simulink model "observer_sim"  (R2020a)
settings: Solver=VariableStepAuto  StartTime=0.0  StopTime=simulation.stopTime  RelTol=1e-3
values from neighbouring files (symbols this model uses):
  L1 = 1    [Main.m]
  L2 = -0.5    [Main.m]
  MaxCrossings = 3    [Main.m]
  TE = 50    [Main.m]
  Threshold = 0.1    [Main.m]
  tp = 1/(2*pi)    (= 0.159154943092)    [Main.m]
undefined symbols (not defined in the file or in its folder): DiscIntNeverNeededParam, servoModel, simulation
libraries: dspsigops x2, mcbcontrolslib x1, simulink x1
settings Model: Creator=FawadFarooq  LastModifiedBy=FawaD KhaN
settings DebuggingCC: SFMachineParentedDataDiag=error

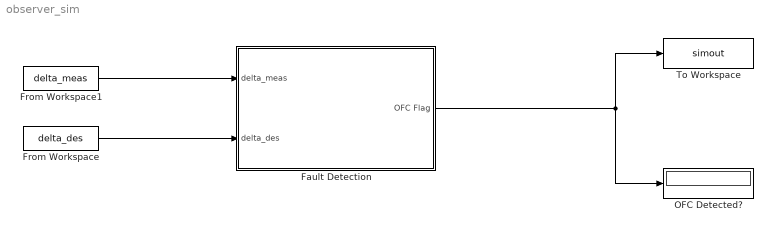
== system observer_sim ==
  Fault Detection : Subsystem
  From Workspace : FromWorkspace  VariableName=delta_des  SampleTime=1/simulation.Fs
  From Workspace1 : FromWorkspace  VariableName=delta_meas  SampleTime=1/simulation.Fs
  OFC Detected? : Display
  To Workspace : ToWorkspace  VariableName=simout  SaveFormat=Timeseries  SampleTime=1/simulation.Fs
  wires:
  Fault Detection/1(OFC Flag) -> OFC Detected?/1, To Workspace/1
  From Workspace1/1 -> Fault Detection/1(delta_meas)
  From Workspace/1 -> Fault Detection/2(delta_des)

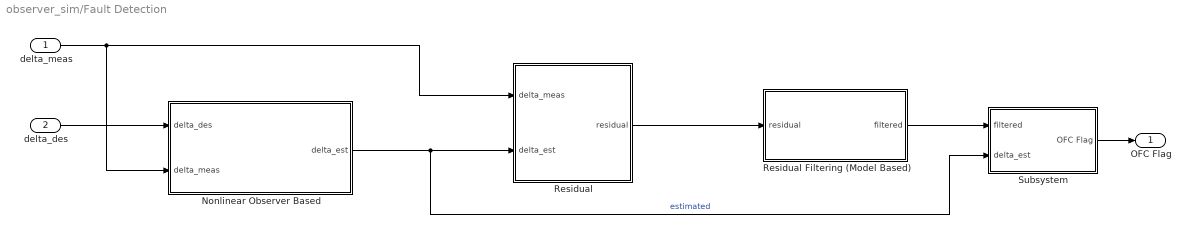
== system observer_sim/Fault Detection ==
  delta_meas : Inport
  delta_des : Inport  Port=2
  Nonlinear Observer Based : Subsystem
  Residual : Subsystem
  Residual Filtering (Model Based) : Subsystem
  Subsystem : Subsystem
  OFC Flag : Outport
  wires:
  Residual/1(residual) -> Residual Filtering (Model Based)/1(residual)
  Nonlinear Observer Based/1(delta_est) -> Subsystem/2(delta_est), Residual/2(delta_est)  "estimated"
  delta_meas/1 -> Nonlinear Observer Based/2(delta_meas), Residual/1(delta_meas)
  Residual Filtering (Model Based)/1(filtered) -> Subsystem/1(filtered)
  delta_des/1 -> Nonlinear Observer Based/1(delta_des)
  Subsystem/1(OFC Flag) -> OFC Flag/1

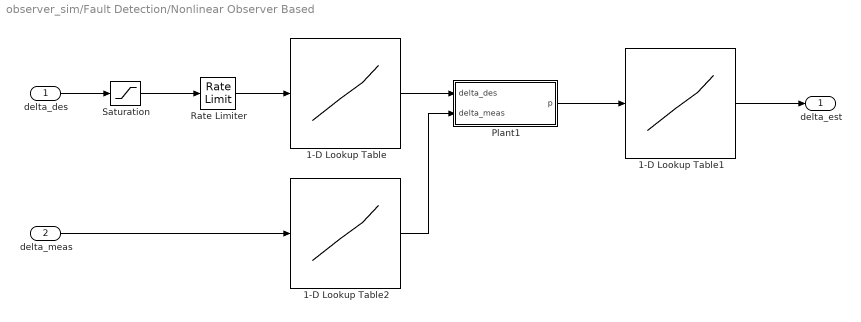
== system observer_sim/Fault Detection/Nonlinear Observer Based ==
  delta_des : Inport
  delta_meas : Inport  Port=2
  1-D Lookup Table : Lookup_n-D  NumberOfTableDimensions=1  BreakpointsForDimension1=[-30,-21,-11,0,14,20]  Table=[77.78,58.55,29.58,0,-37.48,-52.95]  InternalRulePriority=Speed  RndMeth=Simplest  InputSameDT=on
  1-D Lookup Table1 : Lookup_n-D  NumberOfTableDimensions=1  BreakpointsForDimension1=[-52.95, -37.48, 0.0, 29.58, 55.62, 77.78]  Table=[20.0, 14.0, 0.0, -11.0, -21.0, -30.0]  InternalRulePriority=Speed  RndMeth=Simplest  InputSameDT=on
  1-D Lookup Table2 : Lookup_n-D  NumberOfTableDimensions=1  BreakpointsForDimension1=[-30,-21,-11,0,14,20]  Table=[77.78,58.55,29.58,0,-37.48,-52.95]  InternalRulePriority=Speed  RndMeth=Simplest  InputSameDT=on
  Plant1 : Subsystem
  Rate Limiter : RateLimiter  RisingSlewLimit=30  FallingSlewLimit=-30
  Saturation : Saturate  UpperLimit=15  LowerLimit=-30
  delta_est : Outport
  wires:
  Rate Limiter/1 -> 1-D Lookup Table/1
  Saturation/1 -> Rate Limiter/1
  1-D Lookup Table1/1 -> delta_est/1
  delta_des/1 -> Saturation/1
  Plant1/1(p) -> 1-D Lookup Table1/1
  1-D Lookup Table/1 -> Plant1/1(delta_des)
  delta_meas/1 -> 1-D Lookup Table2/1
  1-D Lookup Table2/1 -> Plant1/2(delta_meas)

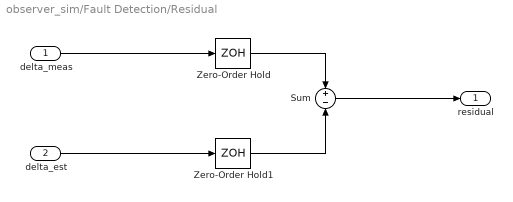
== system observer_sim/Fault Detection/Residual ==
  delta_meas : Inport
  delta_est : Inport  Port=2
  Sum : Sum  Inputs=+|-
  Zero-Order Hold : ZeroOrderHold  SampleTime=1/simulation.Fs
  Zero-Order Hold1 : ZeroOrderHold  SampleTime=1/simulation.Fs
  residual : Outport
  wires:
  Zero-Order Hold/1 -> Sum/1
  delta_meas/1 -> Zero-Order Hold/1
  delta_est/1 -> Zero-Order Hold1/1
  Zero-Order Hold1/1 -> Sum/2
  Sum/1 -> residual/1

== system observer_sim/Fault Detection/Residual Filtering (Model Based) ==
  residual : Inport
  IIR Filter : mcbcontrolslib/IIR Filter  VariantControl=Low Pass Filter  VariantSelect=Low-pass  Filter_constant=0.5  advancedSettings=off  Ts=50e-6  cutOff_freq=3183.0989
      settings: SourceProductBaseCode=MT
  filtered : Outport
  wires:
  IIR Filter/1 -> filtered/1
  residual/1 -> IIR Filter/1

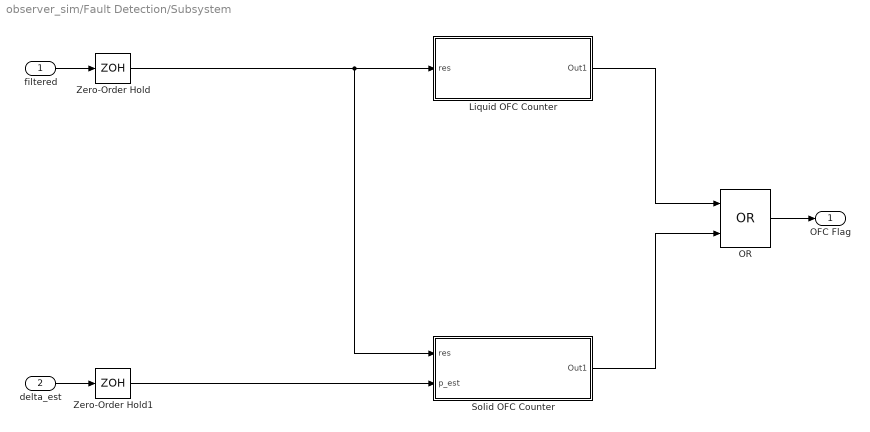
== system observer_sim/Fault Detection/Subsystem ==
  filtered : Inport
  delta_est : Inport  Port=2
  Liquid OFC Counter : Subsystem
  OR : Logic  Operator=OR  IconShape=distinctive  AllPortsSameDT=off  OutDataTypeStr=boolean
  "Solid OFC Counter " : Subsystem
  Zero-Order Hold : ZeroOrderHold  SampleTime=1/simulation.Fs
  Zero-Order Hold1 : ZeroOrderHold  SampleTime=1/simulation.Fs
  OFC Flag : Outport
  wires:
  filtered/1 -> Zero-Order Hold/1
  delta_est/1 -> Zero-Order Hold1/1
  Zero-Order Hold1/1 -> "Solid OFC Counter "/2(p_est)
  Zero-Order Hold/1 -> "Solid OFC Counter "/1(res), Liquid OFC Counter/1(res)
  OR/1 -> OFC Flag/1
  "Solid OFC Counter "/1(Out1) -> OR/2
  Liquid OFC Counter/1(Out1) -> OR/1

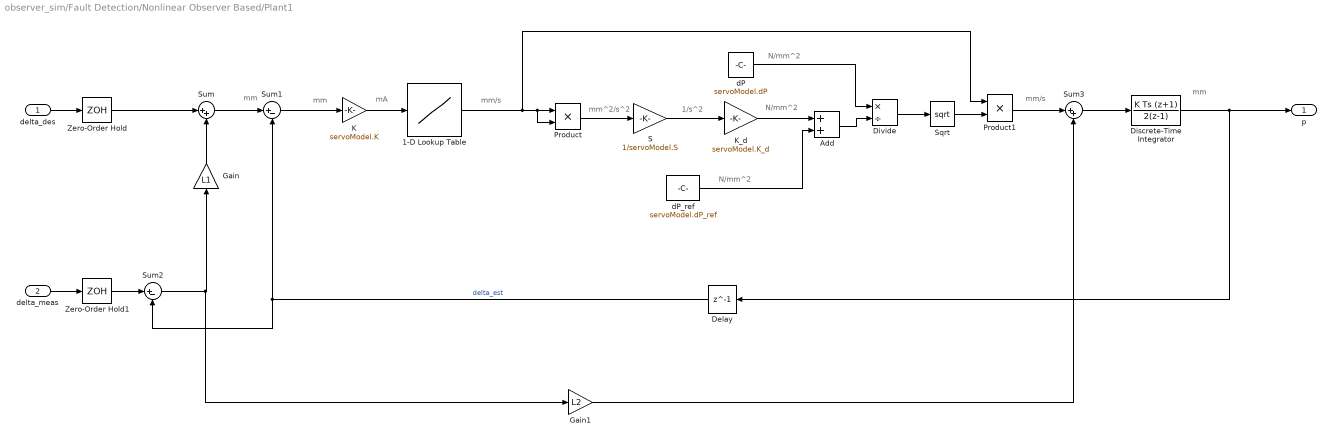
== system observer_sim/Fault Detection/Nonlinear Observer Based/Plant1 ==
  note: N/mm^2
  note: N/mm^2
  note: mm
  note: mA
  note: mm/s
  note: mm^2/s^2
  note: 1/s^2
  note: N/mm^2
  note: mm/s
  note: mm
  note: mm
  delta_des : Inport
  delta_meas : Inport  Port=2
  1-D Lookup Table : Lookup_n-D  NumberOfTableDimensions=1  BreakpointsForDimension1=[-11,-8.45,-2.3,0,2.3,8.45,11]  Table=[-250,-250,-32,0,32,250,250]  InternalRulePriority=Speed  RndMeth=Simplest  InputSameDT=on
  Add : Sum
  Delay : Delay  DelayLength=1  SampleTime=1/simulation.Fs
  Discrete-Time Integrator : DiscreteIntegrator  IntegratorMethod=Integration: Trapezoidal  SampleTime=1/simulation.Fs  ICPrevOutput=DiscIntNeverNeededParam  ICPrevScaledInput=DiscIntNeverNeededParam
  Divide : Product  Inputs=*/
  Gain : Gain  Gain=L1
  Gain1 : Gain  Gain=L2
  K : Gain  Gain=servoModel.K
  K_d : Gain  Gain=servoModel.K_d
  Product : Product
  Product1 : Product
  S : Gain  Gain=1/servoModel.S
  Sqrt : Sqrt  SaturateOnIntegerOverflow=on
  Sum : Sum  Inputs=|++
  Sum1 : Sum  Inputs=|+-
  Sum2 : Sum  Inputs=|+-
  Sum3 : Sum  Inputs=|++
  Zero-Order Hold : ZeroOrderHold  SampleTime=1/simulation.Fs
  Zero-Order Hold1 : ZeroOrderHold  SampleTime=1/simulation.Fs
  dP : Constant  Value=servoModel.dP
  dP_ref : Constant  Value=servoModel.dP_ref
  p : Outport
  wires:
  Delay/1 -> Sum2/2, Sum1/2  "delta_est"
  Discrete-Time Integrator/1 -> p/1, Delay/1
  1-D Lookup Table/1 -> Product1/1, Product/2, Product/1
  dP/1 -> Divide/1
  Sqrt/1 -> Product1/2
  Divide/1 -> Sqrt/1
  S/1 -> K_d/1
  Add/1 -> Divide/2
  K_d/1 -> Add/1
  dP_ref/1 -> Add/2
  Product/1 -> S/1
  K/1 -> 1-D Lookup Table/1
  Sum1/1 -> K/1
  delta_des/1 -> Zero-Order Hold/1
  delta_meas/1 -> Zero-Order Hold1/1
  Zero-Order Hold1/1 -> Sum2/1
  Zero-Order Hold/1 -> Sum/1
  Sum/1 -> Sum1/1
  Gain/1 -> Sum/2
  Product1/1 -> Sum3/1
  Sum3/1 -> Discrete-Time Integrator/1
  Sum2/1 -> Gain1/1, Gain/1
  Gain1/1 -> Sum3/2

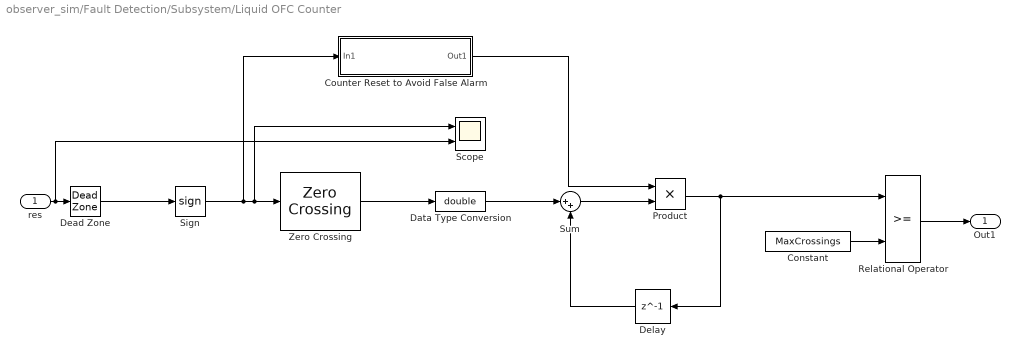
== system observer_sim/Fault Detection/Subsystem/Liquid OFC Counter ==
  res : Inport
  Constant : Constant  Value=MaxCrossings
  Counter Reset to Avoid False Alarm : Subsystem
  Data Type Conversion : DataTypeConversion  OutDataTypeStr=double
  Dead Zone : DeadZone  LowerValue=-Threshold  UpperValue=Threshold  SaturateOnIntegerOverflow=on
  Delay : Delay  DelayLength=1  SampleTime=1/simulation.Fs
  Product : Product
  Relational Operator : RelationalOperator  OutDataTypeStr=boolean  RndMeth=Simplest
  Scope : Scope  NumInputPorts=2
  Sign : Signum
  Sum : Sum  Inputs=|++
  Zero Crossing : dspsigops/Zero Crossing  InputProcessing=Columns as channels (frame based)
      settings: SourceProductBaseCode=DS
  Out1 : Outport
  wires:
  Sum/1 -> Product/2
  Delay/1 -> Sum/2
  Zero Crossing/1 -> Data Type Conversion/1
  Product/1 -> Delay/1, Relational Operator/1
  Relational Operator/1 -> Out1/1
  Sign/1 -> Counter Reset to Avoid False Alarm/1(In1), Scope/1, Zero Crossing/1
  Counter Reset to Avoid False Alarm/1(Out1) -> Product/1
  Dead Zone/1 -> Sign/1
  Data Type Conversion/1 -> Sum/1
  Constant/1 -> Relational Operator/2
  res/1 -> Scope/2, Dead Zone/1

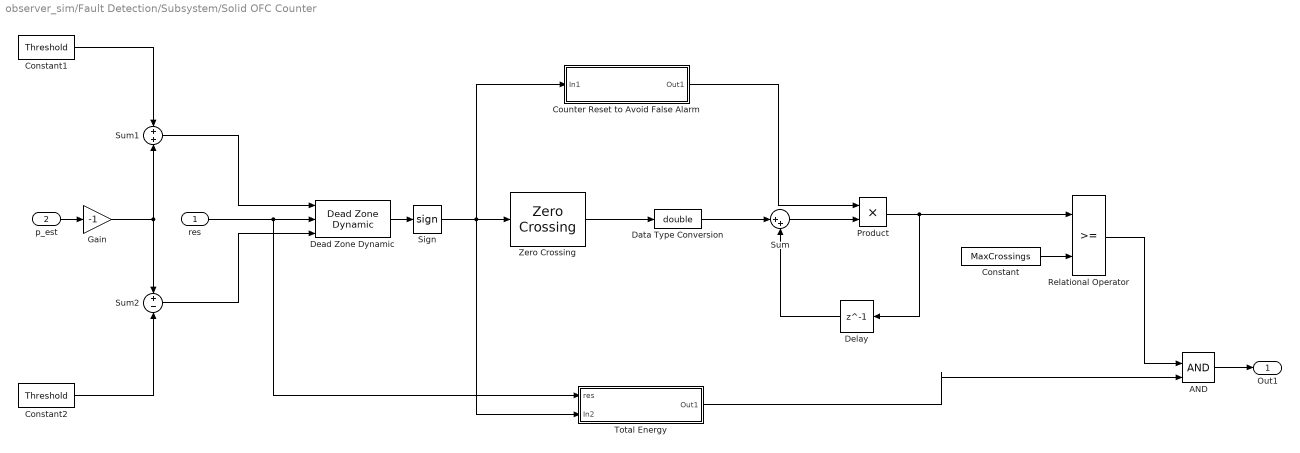
== system observer_sim/Fault Detection/Subsystem/Solid OFC Counter  ==
  res : Inport
  p_est : Inport  Port=2
  AND : Logic  IconShape=distinctive  AllPortsSameDT=off  OutDataTypeStr=boolean
  Constant : Constant  Value=MaxCrossings
  Constant1 : Constant  Value=Threshold
  Constant2 : Constant  Value=Threshold
  Counter Reset to Avoid False Alarm : Subsystem
  Data Type Conversion : DataTypeConversion  OutDataTypeStr=double
  Dead Zone Dynamic : simulink/Discontinuities/Dead Zone Dynamic
      settings: SourceProductBaseCode=SL
  Delay : Delay  DelayLength=1  SampleTime=1/simulation.Fs
  Gain : Gain  Gain=-1
  Product : Product
  Relational Operator : RelationalOperator  OutDataTypeStr=boolean  RndMeth=Simplest
  Sign : Signum
  Sum : Sum  Inputs=|++
  Sum1 : Sum  Inputs=+|+
  Sum2 : Sum  Inputs=+|-
  Total Energy : Subsystem
  Zero Crossing : dspsigops/Zero Crossing  InputProcessing=Columns as channels (frame based)
      settings: SourceProductBaseCode=DS
  Out1 : Outport
  wires:
  p_est/1 -> Gain/1
  Constant/1 -> Relational Operator/2
  Data Type Conversion/1 -> Sum/1
  Dead Zone Dynamic/1 -> Sign/1
  Counter Reset to Avoid False Alarm/1(Out1) -> Product/1
  Sign/1 -> Total Energy/2(In2), Zero Crossing/1, Counter Reset to Avoid False Alarm/1(In1)
  Product/1 -> Relational Operator/1, Delay/1
  Zero Crossing/1 -> Data Type Conversion/1
  Delay/1 -> Sum/2
  Sum/1 -> Product/2
  res/1 -> Total Energy/1(res), Dead Zone Dynamic/2
  Constant1/1 -> Sum1/1
  Constant2/1 -> Sum2/2
  Gain/1 -> Sum1/2, Sum2/1
  Sum1/1 -> Dead Zone Dynamic/1
  Sum2/1 -> Dead Zone Dynamic/3
  Relational Operator/1 -> AND/1
  Total Energy/1(Out1) -> AND/2
  AND/1 -> Out1/1

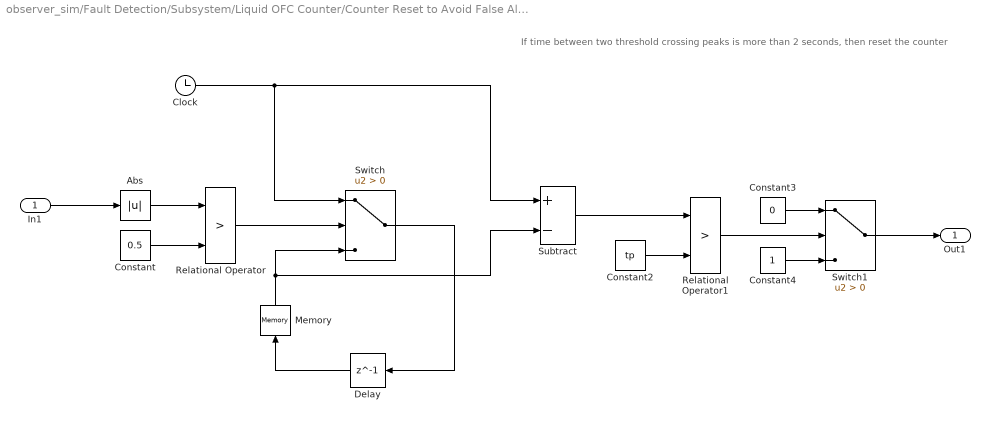
== system observer_sim/Fault Detection/Subsystem/Liquid OFC Counter/Counter Reset to Avoid False Alarm ==
  note: If time between two threshold crossing peaks is more than 2 seconds, then reset the counter
  In1 : Inport
  Abs : Abs
  Clock : Clock
  Constant : Constant  Value=0.5
  Constant2 : Constant  Value=tp
  Constant3 : Constant  Value=0
  Constant4 : Constant
  Delay : Delay  DelayLength=1  SampleTime=1/simulation.Fs
  Memory : Memory
  Relational Operator : RelationalOperator  Operator=>  OutDataTypeStr=boolean  RndMeth=Simplest
  Relational Operator1 : RelationalOperator  Operator=>  OutDataTypeStr=boolean  RndMeth=Simplest
  Subtract : Sum  Inputs=+-
  Switch : Switch  Criteria=u2 > Threshold
  Switch1 : Switch  Criteria=u2 > Threshold
  Out1 : Outport
  wires:
  Switch1/1 -> Out1/1
  In1/1 -> Abs/1
  Abs/1 -> Relational Operator/1
  Constant/1 -> Relational Operator/2
  Relational Operator/1 -> Switch/2
  Switch/1 -> Delay/1
  Delay/1 -> Memory/1
  Memory/1 -> Subtract/2, Switch/3
  Clock/1 -> Subtract/1, Switch/1
  Subtract/1 -> Relational Operator1/1
  Constant2/1 -> Relational Operator1/2
  Relational Operator1/1 -> Switch1/2
  Constant3/1 -> Switch1/1
  Constant4/1 -> Switch1/3

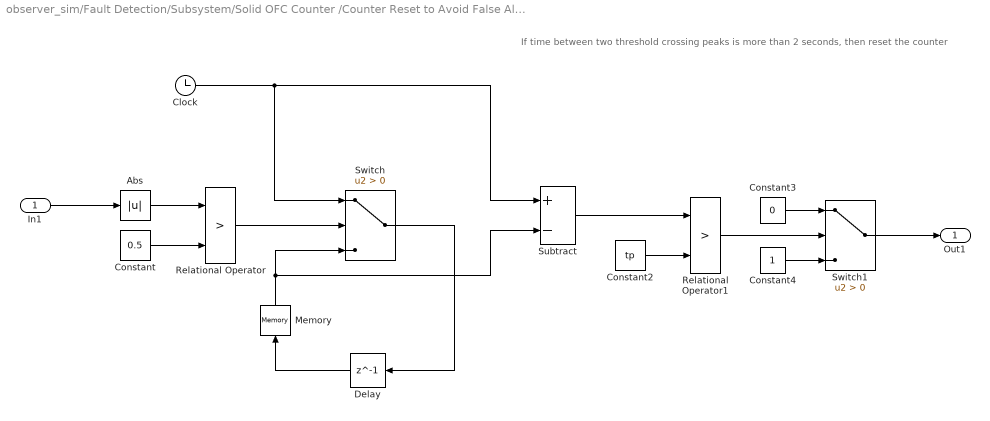
== system observer_sim/Fault Detection/Subsystem/Solid OFC Counter /Counter Reset to Avoid False Alarm ==
  note: If time between two threshold crossing peaks is more than 2 seconds, then reset the counter
  In1 : Inport
  Abs : Abs
  Clock : Clock
  Constant : Constant  Value=0.5
  Constant2 : Constant  Value=tp
  Constant3 : Constant  Value=0
  Constant4 : Constant
  Delay : Delay  DelayLength=1  SampleTime=1/simulation.Fs
  Memory : Memory
  Relational Operator : RelationalOperator  Operator=>  OutDataTypeStr=boolean  RndMeth=Simplest
  Relational Operator1 : RelationalOperator  Operator=>  OutDataTypeStr=boolean  RndMeth=Simplest
  Subtract : Sum  Inputs=+-
  Switch : Switch  Criteria=u2 > Threshold
  Switch1 : Switch  Criteria=u2 > Threshold
  Out1 : Outport
  wires:
  Constant4/1 -> Switch1/3
  Constant3/1 -> Switch1/1
  Relational Operator1/1 -> Switch1/2
  Constant2/1 -> Relational Operator1/2
  Subtract/1 -> Relational Operator1/1
  Clock/1 -> Switch/1, Subtract/1
  Memory/1 -> Switch/3, Subtract/2
  Delay/1 -> Memory/1
  Switch/1 -> Delay/1
  Relational Operator/1 -> Switch/2
  Constant/1 -> Relational Operator/2
  Abs/1 -> Relational Operator/1
  In1/1 -> Abs/1
  Switch1/1 -> Out1/1

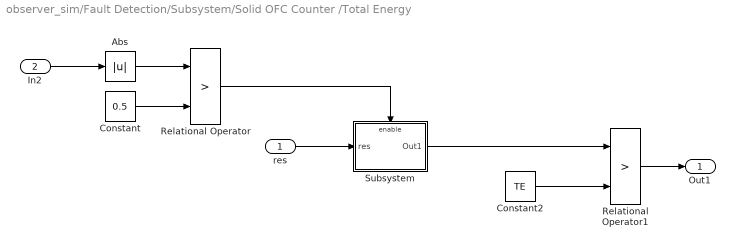
== system observer_sim/Fault Detection/Subsystem/Solid OFC Counter /Total Energy ==
  res : Inport
  In2 : Inport  Port=2
  Abs : Abs
  Constant : Constant  Value=0.5
  Constant2 : Constant  Value=TE
  Relational Operator : RelationalOperator  Operator=>  OutDataTypeStr=boolean  RndMeth=Simplest
  Relational Operator1 : RelationalOperator  Operator=>  OutDataTypeStr=boolean  RndMeth=Simplest
  Subsystem : Subsystem
  Out1 : Outport
  wires:
  Relational Operator1/1 -> Out1/1
  Abs/1 -> Relational Operator/1
  Constant/1 -> Relational Operator/2
  Relational Operator/1 -> Subsystem/Enable
  Constant2/1 -> Relational Operator1/2
  In2/1 -> Abs/1
  res/1 -> Subsystem/1(res)
  Subsystem/1(Out1) -> Relational Operator1/1

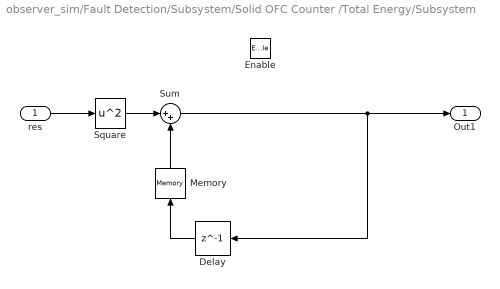
== system observer_sim/Fault Detection/Subsystem/Solid OFC Counter /Total Energy/Subsystem ==
  res : Inport
  Enable : EnablePort  StatesWhenEnabling=reset
  Delay : Delay  DelayLength=1  SampleTime=1/simulation.Fs
  Memory : Memory
  Square : Math  Operator=square  SaturateOnIntegerOverflow=on
  Sum : Sum  Inputs=|++
  Out1 : Outport
  wires:
  res/1 -> Square/1
  Memory/1 -> Sum/2
  Delay/1 -> Memory/1
  Square/1 -> Sum/1
  Sum/1 -> Out1/1, Delay/1
